simulink model "subSystem"  (R2023b)
settings: Solver=VariableStepAuto  StartTime=0.0  StopTime=10.0  RelTol=1e-3
settings Model: Creator=NITRO  LastModifiedBy=NITRO

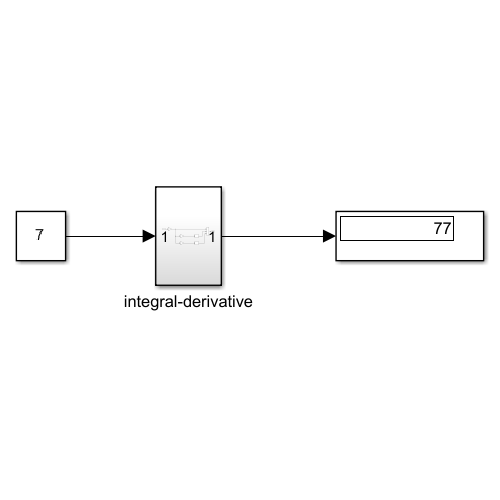
[thumbnail: Simulink's stored preview of the top-level diagram]
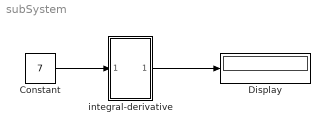
== system subSystem ==
  Constant : Constant  Value=7
  Display : Display
  integral-derivative : Subsystem
  wires:
  Constant/1 -> integral-derivative/1(In1)
  integral-derivative/1(Out1) -> Display/1

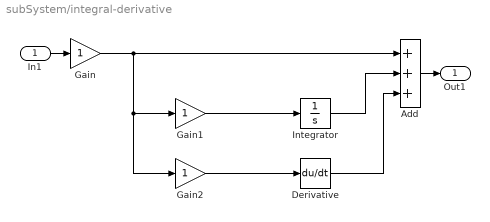
== system subSystem/integral-derivative ==
  In1 : Inport
  Add : Sum  Inputs=+++
  Derivative : Derivative
  Gain : Gain
  Gain1 : Gain
  Gain2 : Gain
  Integrator : Integrator
  Out1 : Outport
  wires:
  Gain2/1 -> Derivative/1
  In1/1 -> Gain/1
  Gain/1 -> Gain2/1, Gain1/1, Add/1
  Derivative/1 -> Add/3
  Gain1/1 -> Integrator/1
  Add/1 -> Out1/1
  Integrator/1 -> Add/2
